simulink model "Ballschuss2"  (Simulink 7.1)
settings: Solver=ode45  StartTime=0.0  StopTime=5  RelTol=1e-3
settings Model: Creator=Meisel  LastModifiedBy=Meisel

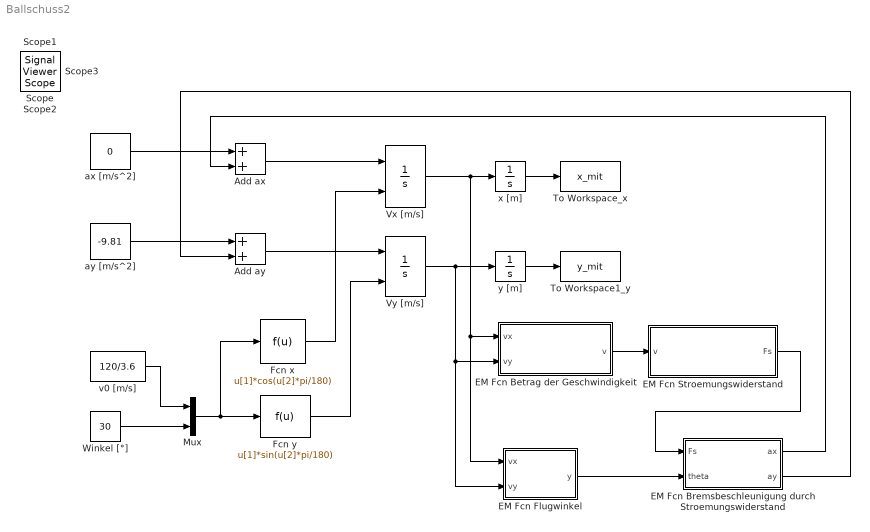
== system Ballschuss2 ==
  Add ax : Sum  OutDataType=sfix(16)  OutScaling=2^-10
  Add ay : Sum  OutDataType=sfix(16)  OutScaling=2^-10
  EM Fcn Betrag der Geschwindigkeit : Stateflow chart
  EM Fcn Bremsbeschleunigung durch Stroemungswiderstand : Stateflow chart
  EM Fcn Flugwinkel : Stateflow chart
  EM Fcn Stroemungswiderstand : Stateflow chart
  Fcn x : Fcn  Expr=u[1]*cos(u[2]*pi/180)
  Fcn y : Fcn  Expr=u[1]*sin(u[2]*pi/180)
  Mux : Mux  Inputs=2
  To Workspace1_y : ToWorkspace  VariableName=y_mit  SampleTime=-1  SaveFormat=Array
  To Workspace_x : ToWorkspace  VariableName=x_mit  SampleTime=-1  SaveFormat=Array
  Vx [m/s] : Integrator  InitialConditionSource=external  InitialCondition=5
  Vy [m/s] : Integrator  InitialConditionSource=external  InitialCondition=5
  Winkel [°] : Constant  Value=30  OutDataType=sfix(16)  OutScaling=2^0
  ax [m/s^2] : Constant  Value=0  OutDataType=sfix(16)  OutScaling=2^0
  ay [m/s^2] : Constant  Value=-9.81  OutDataType=sfix(16)  OutScaling=2^0
  v0 [m/s] : Constant  Value=120/3.6  OutDataType=sfix(16)  OutScaling=2^0
  x [m] : Integrator
  y [m] : Integrator
  Scope{,1..3} (4 alike) : SignalViewerScope  IOType=viewer  RefreshTime=0.035000
      Scope2 settings: SaveName=ScopeData2
      Scope3 settings: SaveName=ScopeData3
  wires:
  Vy [m/s]/1 -> y [m]/1, EM Fcn Betrag der Geschwindigkeit/2(vy), EM Fcn Flugwinkel/2(vy)
  Vx [m/s]/1 -> x [m]/1, EM Fcn Betrag der Geschwindigkeit/1(vx), EM Fcn Flugwinkel/1(vx)
  Winkel [°]/1 -> Mux/2
  Fcn x/1 -> Vx [m/s]/2
  Fcn y/1 -> Vy [m/s]/2
  v0 [m/s]/1 -> Mux/1
  Mux/1 -> Fcn x/1, Fcn y/1
  x [m]/1 -> To Workspace_x/1
  y [m]/1 -> To Workspace1_y/1
  EM Fcn Betrag der Geschwindigkeit/1(v) -> EM Fcn Stroemungswiderstand/1(v)
  EM Fcn Stroemungswiderstand/1(Fs) -> EM Fcn Bremsbeschleunigung durch Stroemungswiderstand/1(Fs)
  EM Fcn Flugwinkel/1(y) -> EM Fcn Bremsbeschleunigung durch Stroemungswiderstand/2(theta)
  ax [m/s^2]/1 -> Add ax/1
  Add ax/1 -> Vx [m/s]/1
  EM Fcn Bremsbeschleunigung durch Stroemungswiderstand/1(ax) -> Add ax/2
  ay [m/s^2]/1 -> Add ay/1
  Add ay/1 -> Vy [m/s]/1
  EM Fcn Bremsbeschleunigung durch Stroemungswiderstand/2(ay) -> Add ay/2

== matlab function EM Fcn Flugwinkel ==
  data: vx input double; y output double; vy input double
function y = Winkel(vx,vy)
y = atan2(vy,vx);

== matlab function EM Fcn Betrag der Geschwindigkeit ==
  data: vx input double; v output double; vy input double
function v = Geschwindigkeit(vx,vy)
v = sqrt(vx*vx+vy*vy);

== matlab function EM Fcn Stroemungswiderstand ==
  data: v input double; Fs output double
function Fs = StroemWidstnd(v)

A   = pi*0.22^2/4; % Flaeche
cw  = 0.25;      % cw-Wert
Rho = 1.29;  % Stoffdichte

Fs = 0.5*v^2*A*cw*Rho;

== matlab function EM Fcn Bremsbeschleunigung durch Stroemungswiderstand ==
  data: Fs input double; ax output double; theta input double; ay output double
function [ax, ay] = aBrems(Fs, theta)

m = 0.45; % 450 g Ballmasse 

Fx = -Fs*cos(theta);
Fy = -Fs*sin(theta);
ax = Fx/m;
ay = Fy/m;
